simulink model "Pipeline_topologies_model"  (R2022b)
settings: Solver=FixedStepAuto  StartTime=0.0  StopTime=t_sim_stop  FixedStep=Ts  RelTol=1e-3
values from neighbouring files (symbols this model uses):
  B = -[1;0;0;0;0;0;0;0;0;0;0;0;0]    [run_pipeline_topologies_model.m]
  B_dem = -[0;0;0;0;0;0;0;0;0;0;0;0;1]    [run_pipeline_topologies_model.m]
  B_h = -[0 0;0 0;0 0;0 0;0 0;1 0;0 0;0 0;0 0;0 0;0 0;0 1;0 0]    [run_pipeline_topologies_model.m]
  c = 330    [run_pipeline_topologies_model.m]
  K_inv = (pi^2)/(64*c^2)*f*D_edge.^5./L_edge    [run_pipeline_topologies_model.m]
  p_init = 0.8*p_eq    [run_pipeline_topologies_model.m]
  V = (pi/8)*sum(((D_edge.^2).*L_edge),2,'omitnan')    [run_pipeline_topologies_model.m]
settings Model: Creator=RASLab-Distributed  LastModifiedBy=RASLab-Distributed

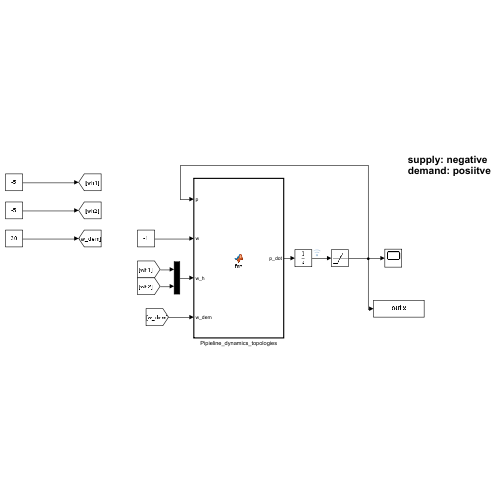
[thumbnail: Simulink's stored preview of the top-level diagram]
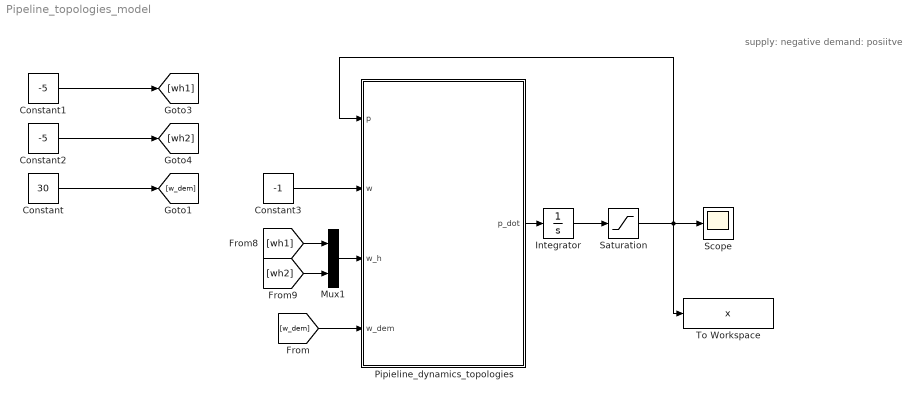
== system Pipeline_topologies_model ==
  note: supply: negative
      | demand: posiitve
  Constant : Constant  Value=30
  Constant1 : Constant  Value=-5
  Constant2 : Constant  Value=-5
  Constant3 : Constant  Value=-1
  Integrator : Integrator  InitialCondition=p_init
  Mux1 : Mux  Inputs=2
  Pipieline_dynamics_topologies : MATLAB Function  TreatAsAtomicUnit=on
  Saturation : Saturate  UpperLimit=inf  LowerLimit=0
  Scope : Scope
  To Workspace : ToWorkspace  VariableName=x  SaveFormat=Timeseries  SampleTime=-1
  wires:
  Pipieline_dynamics_topologies/1(p_dot) -> Integrator/1
  Constant1/1 -> [wh1]
  Constant2/1 -> [wh2]
  Mux1/1 -> Pipieline_dynamics_topologies/3(w_h)
  [wh1] -> Mux1/1
  [wh2] -> Mux1/2
  Constant/1 -> [w_dem]
  [w_dem] -> Pipieline_dynamics_topologies/4(w_dem)
  Constant3/1 -> Pipieline_dynamics_topologies/2(w)
  Integrator/1 -> Saturation/1
  Saturation/1 -> To Workspace/1, Pipieline_dynamics_topologies/1(p), Scope/1

== matlab function Pipeline_topologies_model/Pipieline_dynamics_topologies ==
  data: p input; p_dot output; w input; w_h input; w_dem input; K_inv parameter; c parameter; V parameter; B_h parameter; B_dem parameter; B parameter
function p_dot = fcn(p,w,w_h,w_dem,K_inv, c, V, B_h, B_dem, B)
% COMMENTS HERE

p_sq = p.^2;
l    = ones(length(p),1);  % vector of ones
Psi = sqrt(K_inv.*abs(l*p_sq.' - p_sq*l.')).*sign(l*p.' - p*l.');

p_dot = c^2*(Psi*l)./V + B_h*w_h + B_dem*w_dem + B*w;
